simulink model "processo_fig_7_7_b_NISE_rampa"  (Simulink 8.8)
settings: Solver=VariableStepAuto  StartTime=0.0  StopTime=8  RelTol=1e-3
libraries: simulink x1
settings Model: SuppressorTable=22 serialization::archive 11 0 3 0 0 0 0 0  Creator=fernandopassold  LastModifiedBy=fernandopassold
settings DataIOCC: LimitDataPoints=off  SaveFormat=Dataset  SignalLoggingSaveFormat=Dataset
settings DebuggingCC: UnderspecifiedInitializationDetection=Simplified  MergeDetectMultiDrivingBlocksExec=error  FcnCallInpInsideContextMsg=error  StateNameClashWarn=none  SFUnexpectedBacktrackingDiag=error  SFNoUnconditionalDefaultTransitionDiag=error
settings HardwareCC: ProdBitPerPointer=64  ProdBitPerSizeT=64  ProdBitPerPtrDiffT=64  ProdLargestAtomicFloat=Float  ProdIntDivRoundTo=Zero  ProdEndianess=LittleEndian  ProdWordSize=64  ProdHWDeviceType=Intel->x86-64 (Windows64)
settings ModelReferenceCC: PropagateSignalLabelsOutOfModel=on
settings GRTTargetCC: TargetLangStandard=C99 (ISO)  GeneratePreprocessorConditionals=Use local settings  CombineOutputUpdateFcns=on  GRTInterface=off
settings ConfigComp: CovMetricSettings=dwe  CovHtmlReporting=off  CovSaveCumulativeToWorkspaceVar=off  CovSaveSingleToWorkspaceVar=off  CovExternalEMLEnable=on

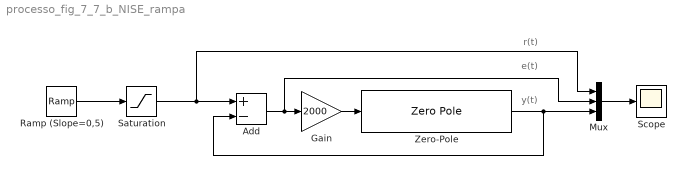
== system processo_fig_7_7_b_NISE_rampa ==
  note: y(t)
  note: e(t)
  note: r(t)
  Add : Sum  Inputs=+-
  Gain : Gain  Gain=2000
  Mux : Mux  Inputs=3
  Ramp (Slope=0,5) : simulink/Sources/Ramp  slope=0.5  start=1  X0=0
  Saturation : Saturate  UpperLimit=2  LowerLimit=0
  Scope : Scope
  Zero-Pole : ZeroPole  Zeros=[-2 -5 -6]  Poles=[0 -8 -10 -12]
  wires:
  Mux/1 -> Scope/1
  Add/1 -> Mux/2, Gain/1
  Gain/1 -> Zero-Pole/1
  Zero-Pole/1 -> Add/2, Mux/3
  Ramp (Slope=0,5)/1 -> Saturation/1
  Saturation/1 -> Mux/1, Add/1
